simulink model "PubIfControlLATC_MDL_DS"  (R2020b)
settings: configuration reference "DspaceConfig" (kept outside this file)
PostLoadFcn:
  | if any(exist('dsrtsu_mdlpostloadfcn', 'file') ~= 0), dsrtsu_mdlpostloadfcn('Execute', bdroot); end
InitFcn:
  | , if any(exist('rtifpga_mdlclblib', 'file') ~= 0), rtifpga_mdlclblib('Init', bdroot); end,
  | , if any(exist('dsmpb_private', 'file') ~= 0), dsmpb_private('dsmpb_mdlclblib', 'Init', bdroot); end,
undefined symbols (not defined in the file): EPS_DrvInpTrqVal_HighReslolution, EPS_LKATorqOvrlDlvd, EPS_LKATorqOvrlDlvdVld, SteerWheelAng, SteerWheelAngSign, SteerWheelSpd, SteerWheelSpdSign
PreSaveFcn:
  | , if any(exist('dsmpb_private', 'file') ~= 0), dsmpb_private('dsmpb_mdlclblib', 'PreSave', bdroot); end,
CloseFcn:
  | , if any(exist('dsmpb_private', 'file') ~= 0), dsmpb_private('dsmpb_mdlclblib', 'Close', bdroot); end,
settings Model: DataDictionary=LCS_v05.sldd  RTICANMMDATA=struct('GeneralSetupData',struct('modelroot','C:\Users\GW00133806\Desktop\ADAS_Store\Adas\LATC','generalsettings',struct('filesettings',struct('destfolder',struct('Name','RTICANMM_FILES','Check',1),'buildfolder',struct('Name','.','Check',1),'AbsDestfolder',struct('Name','C:\Users\GW00133806\Desktop\ADAS_Store\Adas\LATC\RTICANMM_FILES'),'AbsBuildfolder',struct('Name','C:\Users\GW00133806\Desktop\ADAS_Store\Adas\LATC'))),'options',struct('addpaths',1,'rmpaths',1,'addtrcexclusion',false,'cannavigator',struct('checkmonitoring',0),'show_usrtrc',0,'use_usrtrc',0),'advanced',struct('options',ones(1,100)),'MPSetup',{{}},'RTI',struct('Type','DSRT','Ver','4.4','Date','02-Nov-2020'),'modelname','PubIfControlLATC_MDL','block','PubIfControlLATC_MDL'))  DSRTSU_INTERNAL_RTIFPGA=170  DSMPB_ID_DATA={}  OrderedModelArguments=off  Creator=GW00180895
settings ConfigSetRef: SourceName=DspaceConfig

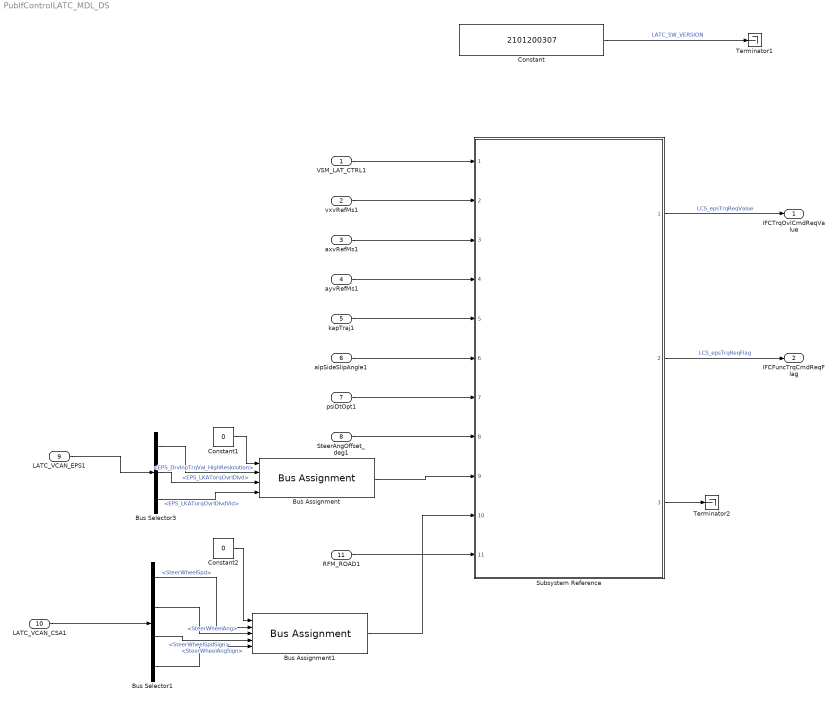
== system PubIfControlLATC_MDL_DS ==
  VSM_LAT_CTRL1 : Inport  OutDataTypeStr=Bus: VSM_LAT_CTRL_BUS  PortDimensions=1  Interpolate=off  BusOutputAsStruct=on
  vxvRefMs1 : Inport  Port=2  OutDataTypeStr=single  PortDimensions=1  Interpolate=off  BusOutputAsStruct=on
  axvRefMs1 : Inport  Port=3  OutDataTypeStr=single  PortDimensions=1  Interpolate=off  BusOutputAsStruct=on
  ayvRefMs1 : Inport  Port=4  OutDataTypeStr=single  PortDimensions=1  Interpolate=off  BusOutputAsStruct=on
  kapTraj1 : Inport  Port=5  OutDataTypeStr=single  PortDimensions=1  Interpolate=off  BusOutputAsStruct=on
  alpSideSlipAngle1 : Inport  Port=6  OutDataTypeStr=single  PortDimensions=1  Interpolate=off  BusOutputAsStruct=on
  psiDtOpt1 : Inport  Port=7  OutDataTypeStr=single  PortDimensions=1  Interpolate=off  BusOutputAsStruct=on
  SteerAngOffset_deg1 : Inport  Port=8  OutDataTypeStr=single  PortDimensions=1  Interpolate=off  BusOutputAsStruct=on
  LATC_VCAN_EPS1 : Inport  Port=9  OutDataTypeStr=Bus: LATC_VCAN_EPS_BUS  PortDimensions=1  Interpolate=off  BusOutputAsStruct=on
  LATC_VCAN_CSA1 : Inport  Port=10  OutDataTypeStr=Bus: LATC_VCAN_CSA_BUS  PortDimensions=1  Interpolate=off  BusOutputAsStruct=on
  RFM_ROAD1 : Inport  Port=11  OutDataTypeStr=Bus: RFM_ROAD_BUS  PortDimensions=1  Interpolate=off  BusOutputAsStruct=on
  Bus Assignment : BusAssignment  AssignedSignals=EPS_DrvInpTrqVal_HighReslolution,EPS_LKATorqOvrlDlvd,EPS_LKATorqOvrlDlvdVld
  Bus Assignment1 : BusAssignment  AssignedSignals=SteerWheelSpd,SteerWheelAng,SteerWheelSpdSign,SteerWheelAngSign
  Bus Selector1 : BusSelector  OutputSignals=SteerWheelSpd,SteerWheelAng,SteerWheelSpdSign,SteerWheelAngSign
  Bus Selector3 : BusSelector  OutputSignals=EPS_DrvInpTrqVal_HighReslolution,EPS_LKATorqOvrlDlvd,EPS_LKATorqOvrlDlvdVld
  Constant : Constant  Value=2101200307  OutDataTypeStr=uint32
  Constant1 : Constant  Value=0  OutDataTypeStr=Bus: VCAN_EPS_MSG_BUS
  Constant2 : Constant  Value=0  OutDataTypeStr=Bus: VCAN_CSA_MSG_BUS
  Subsystem Reference : Subsystem  ReferencedSubsystem=PvtSubSys_LATC
  Terminator1 : Terminator
  Terminator2 : Terminator
  IFCTrqOvlCmdReqValue : Outport  OutDataTypeStr=single  PortDimensions=1  BusOutputAsStruct=on
  IFCFuncTrqCmdReqFlag : Outport  Port=2  OutDataTypeStr=uint8  PortDimensions=1  BusOutputAsStruct=on
  wires:
  alpSideSlipAngle1/1 -> Subsystem Reference/6
  Subsystem Reference/1 -> IFCTrqOvlCmdReqValue/1  "LCS_epsTrqReqValue"
  ayvRefMs1/1 -> Subsystem Reference/4
  Bus Assignment/1 -> Subsystem Reference/9
  axvRefMs1/1 -> Subsystem Reference/3
  RFM_ROAD1/1 -> Subsystem Reference/11
  kapTraj1/1 -> Subsystem Reference/5
  Subsystem Reference/2 -> IFCFuncTrqCmdReqFlag/1  "LCS_epsTrqReqFlag"
  psiDtOpt1/1 -> Subsystem Reference/7
  VSM_LAT_CTRL1/1 -> Subsystem Reference/1
  Bus Assignment1/1 -> Subsystem Reference/10
  vxvRefMs1/1 -> Subsystem Reference/2
  SteerAngOffset_deg1/1 -> Subsystem Reference/8
  Constant/1 -> Terminator1/1  "LATC_SW_VERSION"
  Subsystem Reference/3 -> Terminator2/1
  Constant1/1 -> Bus Assignment/1
  LATC_VCAN_EPS1/1 -> Bus Selector3/1
  Bus Selector3/1 -> Bus Assignment/2  "<EPS_DrvInpTrqVal_HighReslolution>"
  Bus Selector3/2 -> Bus Assignment/3  "<EPS_LKATorqOvrlDlvd>"
  Bus Selector3/3 -> Bus Assignment/4  "<EPS_LKATorqOvrlDlvdVld>"
  LATC_VCAN_CSA1/1 -> Bus Selector1/1
  Constant2/1 -> Bus Assignment1/1
  Bus Selector1/3 -> Bus Assignment1/4  "<SteerWheelSpdSign>"
  Bus Selector1/4 -> Bus Assignment1/5  "<SteerWheelAngSign>"
  Bus Selector1/2 -> Bus Assignment1/3  "<SteerWheelAng>"
  Bus Selector1/1 -> Bus Assignment1/2  "<SteerWheelSpd>"
